simulink model "sim_disc"  (R2022a)
settings: Solver=VariableStepAuto  StartTime=0.0  StopTime=60  MaxStep=0.001  RelTol=1e-3
undefined symbols (not defined in the file): Discrete, dt, lim_U, msys, sigmas, Time
libraries: cstblocks x2, ctrlSharedLib x1
settings Model: Creator=Rafael  LastModifiedBy=Rafael

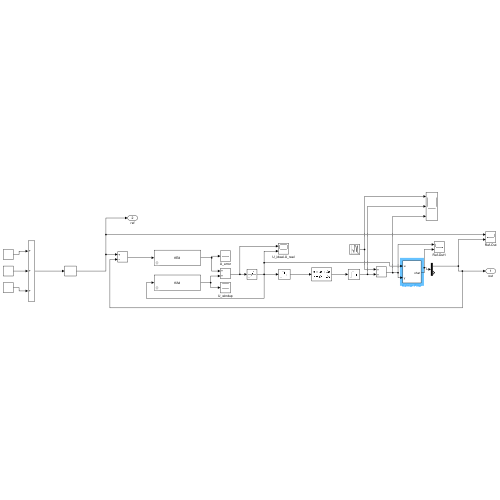
[thumbnail: Simulink's stored preview of the top-level diagram]
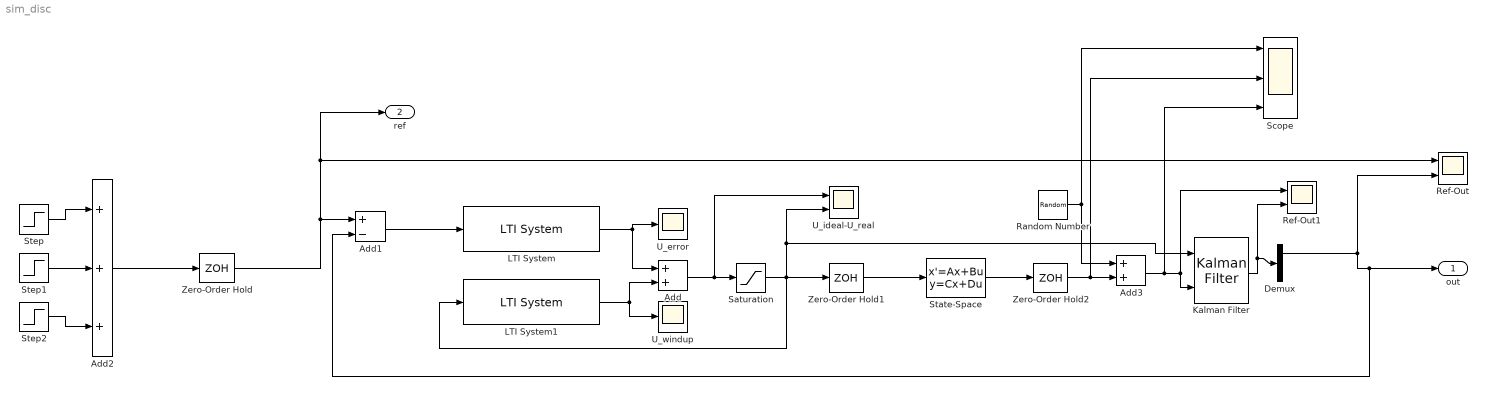
== system sim_disc ==
  Add : Sum
  Add1 : Sum  Inputs=+-
  Add2 : Sum  Inputs=+++
  Add3 : Sum
  Demux : Demux  Outputs=2
  Kalman Filter : ctrlSharedLib/Kalman Filter  TimeDomain=Discrete-Time  UseCurrentEstimator=on  ModelSource=Individual A, B, C, D matrices  ModelSourceVariable=ss(0.95,1,1,0,1)  A=msys{4}.A  B=msys{4}.B  C=msys{4}.C  D=msys{4}.D  NumberOfStates=1  NumberOfInputs=1  NumberOfOutputs=1  InitialEstimateSource=Dialog  X0=0  P0=10  UseK=off  UseGH=off  NumberOfProcessNoiseInputs=1  G=1  TimeInvariantG=on  H=0  TimeInvariantH=on  Q=1  TimeInvariantQ=on  R=max(sigmas').^2  TimeInvariantR=on  N=0  TimeInvariantN=on  AddInputPort=on  AddEnablePort=off  OutputEstimatedY=off  OutputP=off  Ts=dt
  LTI System : cstblocks/LTI System  sys=tfEd  IC=[]
  LTI System1 : cstblocks/LTI System  sys=tfAd  IC=[]
  Random Number : RandomNumber  Variance=max(sigmas').^2  Seed=300  SampleTime=dt
  Ref-Out : Scope  NumInputPorts=2
  Ref-Out1 : Scope  NumInputPorts=2
  Saturation : Saturate  UpperLimit=lim_U  LowerLimit=-lim_U
  Scope : Scope  NumInputPorts=3
  State-Space : StateSpace  A=msys{j}.A  B=msys{j}.B  C=msys{j}.C  D=msys{j}.D  InitialCondition=0
  Step : Step  Time=5  SampleTime=0
  Step1 : Step  Time=20  After=20  SampleTime=0
  Step2 : Step  Time=40  After=-10  SampleTime=0
  U_error : Scope
  U_ideal-U_real : Scope  NumInputPorts=2
  U_windup : Scope
  Zero-Order Hold : ZeroOrderHold  SampleTime=dt
  Zero-Order Hold1 : ZeroOrderHold  SampleTime=dt
  Zero-Order Hold2 : ZeroOrderHold  SampleTime=dt
  out : Outport
  ref : Outport  Port=2
  wires:
  State-Space/1 -> Zero-Order Hold2/1
  Add/1 -> U_ideal-U_real/1, Saturation/1
  LTI System/1 -> Add/1, U_error/1
  LTI System1/1 -> U_windup/1, Add/2
  Demux/1 -> out/1, Add1/2, Ref-Out/2
  Add1/1 -> LTI System/1
  Add2/1 -> Zero-Order Hold/1
  Saturation/1 -> Zero-Order Hold1/1, U_ideal-U_real/2, Kalman Filter/1, LTI System1/1
  Step/1 -> Add2/1
  Step1/1 -> Add2/2
  Step2/1 -> Add2/3
  Zero-Order Hold/1 -> ref/1, Ref-Out/1, Add1/1
  Zero-Order Hold1/1 -> State-Space/1
  Add3/1 -> Scope/3, Ref-Out1/1, Kalman Filter/2
  Kalman Filter/1 -> Ref-Out1/2, Demux/1
  Random Number/1 -> Add3/1, Scope/1
  Zero-Order Hold2/1 -> Scope/2, Add3/2
